simulink model "BERNABE_UNIGO_PROBLEM1"  (R2023b)
settings: Solver=VariableStepAuto  StartTime=0.0  StopTime=20  RelTol=1e-3
values from neighbouring files (symbols this model uses):
  G1_den = [1 0 0]    [BERNABE_UNIGO_NUMBER1.m]    (also in LANDICHO_MACARAIG_NUMBER 2.m)
  G1_num = [1]    [BERNABE_UNIGO_NUMBER1.m]    (also in LANDICHO_MACARAIG_NUMBER 2.m = 1)
  G2_den = [1 1]    [BERNABE_UNIGO_NUMBER1.m]    (also in LANDICHO_MACARAIG_NUMBER 2.m)
  G2_num = [1]    [BERNABE_UNIGO_NUMBER1.m]    (also in LANDICHO_MACARAIG_NUMBER 2.m = 1)
  G3_den = [1 0]    [BERNABE_UNIGO_NUMBER1.m]    (also in LANDICHO_MACARAIG_NUMBER 2.m)
  G3_num = [1]    [BERNABE_UNIGO_NUMBER1.m]    (also in LANDICHO_MACARAIG_NUMBER 2.m = 1)
  H1_den = [1 0]    [BERNABE_UNIGO_NUMBER1.m]    (also in LANDICHO_MACARAIG_NUMBER 2.m)
  H1_num = [1]    [BERNABE_UNIGO_NUMBER1.m]    (also in LANDICHO_MACARAIG_NUMBER 2.m = 1)
  H2_den = [1 -1]    [BERNABE_UNIGO_NUMBER1.m]    (also in LANDICHO_MACARAIG_NUMBER 2.m)
  H2_num = [1]    [BERNABE_UNIGO_NUMBER1.m]    (also in LANDICHO_MACARAIG_NUMBER 2.m = 1)
  H3_den = [1 -2]    [BERNABE_UNIGO_NUMBER1.m]    (also in LANDICHO_MACARAIG_NUMBER 2.m)
  H3_num = [1]    [BERNABE_UNIGO_NUMBER1.m]    (also in LANDICHO_MACARAIG_NUMBER 2.m = 1)
  TF_den = conv(TF4_den,TF6_den)    [BERNABE_UNIGO_NUMBER1.m]
  TF_num = conv(TF4_num,TF6_num)    [BERNABE_UNIGO_NUMBER1.m]
settings Model: Creator=ACER  LastModifiedBy=user

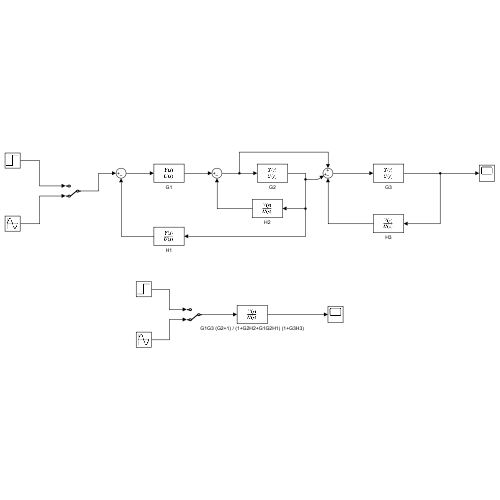
[thumbnail: Simulink's stored preview of the top-level diagram]
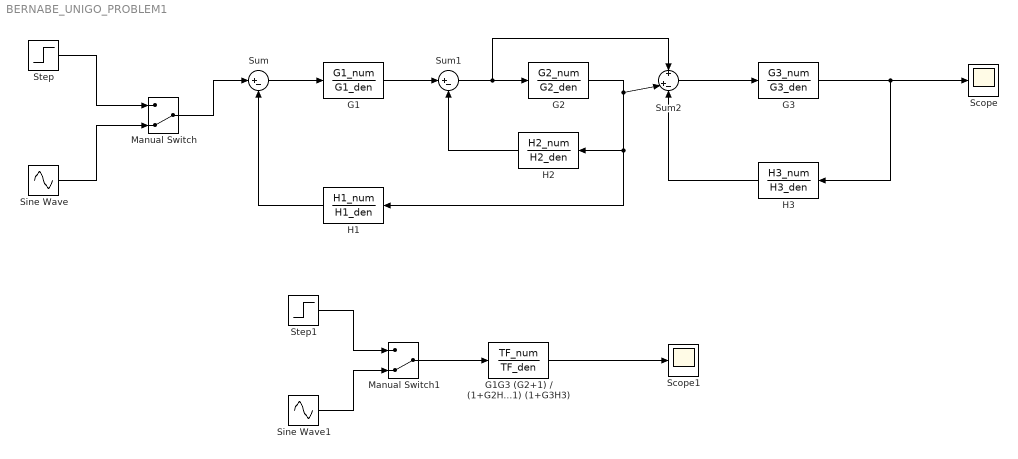
== system BERNABE_UNIGO_PROBLEM1 ==
  G1 : TransferFcn  Numerator=G1_num  Denominator=G1_den
  G1G3 (G2+1) / (1+G2H2+G1G2H1) (1+G3H3) : TransferFcn  Numerator=TF_num  Denominator=TF_den
  G2 : TransferFcn  Numerator=G2_num  Denominator=G2_den
  G3 : TransferFcn  Numerator=G3_num  Denominator=G3_den
  H1 : TransferFcn  Numerator=H1_num  Denominator=H1_den
  H2 : TransferFcn  Numerator=H2_num  Denominator=H2_den
  H3 : TransferFcn  Numerator=H3_num  Denominator=H3_den
  Manual Switch : ManualSwitch  CurrentSetting=0
  Manual Switch1 : ManualSwitch  CurrentSetting=0
  Scope : Scope
  Scope1 : Scope
  Sine Wave : Sin  SampleTime=0
  Sine Wave1 : Sin  SampleTime=0
  Step : Step  Time=0  SampleTime=0
  Step1 : Step  Time=0  SampleTime=0
  Sum : Sum  Inputs=|+-
  Sum1 : Sum  Inputs=|+-
  Sum2 : Sum  Inputs=+|+-
  wires:
  H3/1 -> Sum2/3
  H2/1 -> Sum1/2
  G1G3 (G2+1) / (1+G2H2+G1G2H1) (1+G3H3)/1 -> Scope1/1
  Sum2/1 -> G3/1
  G1/1 -> Sum1/1
  G2/1 -> H1/1, H2/1, Sum2/2
  G3/1 -> H3/1, Scope/1
  Sum1/1 -> G2/1, Sum2/1
  Sum/1 -> G1/1
  H1/1 -> Sum/2
  Step/1 -> Manual Switch/1
  Sine Wave/1 -> Manual Switch/2
  Manual Switch/1 -> Sum/1
  Manual Switch1/1 -> G1G3 (G2+1) / (1+G2H2+G1G2H1) (1+G3H3)/1
  Step1/1 -> Manual Switch1/1
  Sine Wave1/1 -> Manual Switch1/2
